simulink model "Biped_Model"  (R2019a)
settings: Solver=VariableStepAuto  StartTime=0.0  StopTime=Time(end)  FixedStep=.001  EnableMultiTasking=on
PreLoadFcn:
  | YBT_HomeDir = pwd;
  | 
  | % Code to use copy within this repository
  | addpath([YBT_HomeDir filesep 'Libraries' filesep 'CFL_Libs']);
  | startup_Contact_Forces
  | 
  | cd(YBT_HomeDir)
  | addpath(YBT_HomeDir);
  | addpath([YBT_HomeDir filesep 'Libraries']);
  | addpath([YBT_HomeDir filesep 'Images']);
  | 
  | Robot_Parameters
model workspace: external: MATLAB File C:\Users\nozaripo\Desktop\BipedalWalking_Simulink_ModelnData\Robot_Parameters.m (data not in the file)
values from neighbouring files (symbols this model uses):
  ankle_servo_kd = 4    [Robot_Parameters.m]
  ankle_servo_ki = 0    [Robot_Parameters.m]
  ankle_servo_kp = 70    [Robot_Parameters.m]
  ankle_to_midLow = 19    [Robot_Parameters.m]
  contact_damping = 50    [Robot_Parameters.m]
  contact_point_radius = 0.005    [Robot_Parameters.m]
  contact_stiffness = 90311    [Robot_Parameters.m]
  deriv_filter_coeff = 50    [Robot_Parameters.m]
  foot_mass = 1    [Robot_Parameters.m]
  height_plane = 0.1    [Robot_Parameters.m]
  hip_servo_kd = 30    [Robot_Parameters.m]
  hip_servo_ki = 0    [Robot_Parameters.m]
  hip_servo_kp = 300    [Robot_Parameters.m]
  init = -joint_angles(1,:)    [Script_Data.m]
  init_vel = -vel(1,:)    [Script_Data.m]
  joint_angles = joint_angles(:,end:-1:1)    [Script_Data.m]
  joint_damping = 0    [Robot_Parameters.m]
  joint_stiffness = 0    [Robot_Parameters.m]
  knee_servo_kd = 30    [Robot_Parameters.m]
  knee_servo_ki = 0    [Robot_Parameters.m]
  knee_servo_kp = 150    [Robot_Parameters.m]
  knee_to_midUpp = 19    [Robot_Parameters.m]
  linear_contact_flag = 0    [Robot_Parameters.m]
  lower_leg_CM_offset = 2.55    [Robot_Parameters.m]
  lower_leg_mass = 2.87    [Robot_Parameters.m]
  max_torque_ank = 45    [Robot_Parameters.m]
  max_torque_hip = 25    [Robot_Parameters.m]
  max_torque_kn = 30    [Robot_Parameters.m]
  midLow_to_knee = 19    [Robot_Parameters.m]
  midUpp_to_hip = 19    [Robot_Parameters.m]
  motion_time_constant = 0.01    [Robot_Parameters.m]
  motor_constant = 0.01    [Robot_Parameters.m]
  motor_inertia = 0    [Robot_Parameters.m]
  mu_k = 0.5    [Robot_Parameters.m]
  mu_s = 0.8    [Robot_Parameters.m]
  mu_vth = 0.1    [Robot_Parameters.m]
  pen_exp = 1.5    [Robot_Parameters.m]
  plane_x = 3    [Robot_Parameters.m]
  plane_y = 0.3    [Robot_Parameters.m]
  split_belt = 0    [Script_Data.m]
  Time = (0:.01:.01*209)'    [Script_Data.m]
  torso_mass = 27.17    [Robot_Parameters.m]
  torso_to_hip = 11    [Robot_Parameters.m]
  upper_leg_CM_offset = 2.55    [Robot_Parameters.m]
  upper_leg_length = 38    [Robot_Parameters.m]
  upper_leg_mass = 4.7    [Robot_Parameters.m]
  V_treadmill = -1.0    (= -1)    [Script_Data.m]
  YBT_Par = struct    [Robot_Parameters.m]
undefined symbols (not defined in the file or in its folder): Extr_Data_LinkHoles, X, Y, Z
libraries: nesl_utility x198, sm_lib x144, fl_lib x42, simulink x20, ee_lib x18, Contact_Forces_Lib x16, Parts_Lib x10, Multibody_Multiphysics_Lib x6, simulink_extras x1
(part 11 of 11)

== system Biped_Model/Robot/Robot Leg L/Box to Belt In Force1/Sphere to Plane Force Enabled nz1/Forces/Force Law ==
  note: 1) Only subsystems can be added as variant choices at this level
      | 2) Blocks cannot be connected at this level as connectivity is
      | automatically determined at simulation, based on the active variant
  Pen : Inport
  Pen Vel : Inport  Port=2
  Custom : Subsystem  VariantControl=Custom  mask(Custom Force Law){k_pen=k_contact, b_penvel=b_contact, cust_param_1=custom_param_1, cust_param_2=custom_param_2}
      mask prompts: k_pen "Contact Stiffness"; b_penvel "Contact Damping"; cust_param_1 "Custom Parameter 1"; cust_param_2 "Custom Parameter 2"
      mask help: This subsystem is for prototyping a custom force law. You can create your own force law in this subsystem and use it in the contact force models in this library by selecting the "Custom" option for the Force Law parameter.
  Linear : Subsystem  VariantControl=Linear  mask(Linear Force Law){k_pen=k_contact, b_penvel=b_contact}
      mask prompts: k_pen "Contact Stiffness"; b_penvel "Contact Damping"
      mask help: Implements a contact force law as a linear spring damper. The damping force is applied only as the penetration depth increases.
      mask Help: web(which('Force_Laws.html'));
  Nonlinear : Subsystem  VariantControl=Nonlinear  mask(Nonlinear Force Law){k_pen=k_contact, b_penvel=b_contact, pen_full_damping=pen_full_damp_F, pen_exp=pen_exponent}
      mask prompts: k_pen "Contact Stiffness"; b_penvel "Contact Damping"; pen_full_damping "Penetration for Full Damping"; pen_exp "Penetration Exponent (>=1)"
      mask help: Implements a contact force law as a nonlinear spring damper. The spring force increases exponentially with penetration. The damping force is multiplied by a scaling factor which is dependent upon the penetration. The scaling factor increases from 0 to 1 as a smooth polynomial until the penetration reaches the value specified by the parameter Penetration for Full Damping. The damping force is applied only as the penetration depth increases.
      mask Help: web(which('Force_Laws.html'));
  Spr F : Outport
  Damp F : Outport  Port=2

== system Biped_Model/Robot/Robot Leg L/Box to Belt In Force1/Sphere to Plane Force Enabled nz2/Forces/Calculate Penetration ==
  z : Inport
  vz : Inport  Port=2
  Abs : Abs  ZeroCross=off
  Constant : Constant  Value=sphere_rad+plane_depth
  Dead Zone : DeadZone  LowerValue=-inf  UpperValue=0  SaturateOnIntegerOverflow=on
  Gain2 : Gain  Gain=-1
  Product : Product
  Sign vx : Signum  ZeroCross=off
  Sign x : Signum  ZeroCross=off
  Sum : Sum  Inputs=+-
  Pos Sign : Outport
  Pen : Outport  Port=2
  Pen Vel : Outport  Port=3
  Vel Sign : Outport  Port=4
  wires:
  Gain2/1 -> Pen Vel/1
  Dead Zone/1 -> Pen/1
  Product/1 -> Gain2/1
  Sign vx/1 -> Vel Sign/1
  Sign x/1 -> Product/1, Pos Sign/1
  Abs/1 -> Sum/2
  Sum/1 -> Dead Zone/1
  Constant/1 -> Sum/1
  vz/1 -> Sign vx/1, Product/2
  z/1 -> Abs/1, Sign x/1

== system Biped_Model/Robot/Robot Leg L/Box to Belt In Force1/Sphere to Plane Force Enabled nz2/Forces/Ff ==
  Fn : Inport
  R : Inport  Port=2
  zSign : Inport  Port=3
  wx : Inport  Port=4
  wy : Inport  Port=5
  vx : Inport  Port=6
  vy : Inport  Port=7
  Cross Product : Contact_Forces_Lib/Math/Cross Product  SystemSampleTime=-1
      settings: SourceProductName=Simscape Multibody Contact Forces Library
  Friction Law : Contact_Forces_Lib/Friction Law  SystemSampleTime=-1  LabelModeActiveChoice=Stick_Slip_C
      settings: SourceProductName=Simscape Multibody Contact Forces Library
  Fx1 : Constant  Value=0
  Fx2 : Constant  Value=[0 0 -sphere_rad]
  Gain : Gain  Gain=-1
  Mux1 : Mux  Inputs=3
  Product1 : Product  Inputs=/*  Multiplication=Matrix(*)
  Product2 : Product  Inputs=/*  Multiplication=Matrix(*)
  Product{3..7} (5 alike) : Product
  Selector : Selector  InputPortWidth=3  IndexOptions=Index vector (dialog)  Indices=3  OutputSizes=1
  SlipVel : Subsystem
  Trigonometric Function : Trigonometry
  Trigonometric Function1 : Trigonometry  Operator=cos
  zSign1 : InportShadow  Port=3
  Ff Sph : Outport
  T Sph : Outport  Port=2
  Ff Pla : Outport  Port=3
  wires:
  Product7/1 -> Cross Product/1
  zSign1/1 -> Product7/2
  Product6/1 -> SlipVel/3(vx)
  zSign/1 -> Product6/2, Product5/1
  Product5/1 -> SlipVel/4(vy)
  Fx2/1 -> Product7/1
  R/1 -> Product2/1, Product1/1
  Cross Product/1 -> Product2/2
  Product1/1 -> Ff Sph/1
  Mux1/1 -> Product1/2, Cross Product/2, Gain/1
  Product2/1 -> T Sph/1
  vy/1 -> Product5/2
  wy/1 -> SlipVel/2(wy)
  wx/1 -> SlipVel/1(wx)
  vx/1 -> Product6/1
  Trigonometric Function/1 -> Product4/2
  Fx1/1 -> Mux1/3
  Product3/1 -> Mux1/1
  Product4/1 -> Mux1/2
  Friction Law/1 -> Product4/1, Product3/1
  Selector/1 -> Friction Law/1
  SlipVel/1(vabs) -> Friction Law/2
  Trigonometric Function1/1 -> Product3/2
  SlipVel/2(alpha) -> Trigonometric Function1/1, Trigonometric Function/1
  Gain/1 -> Ff Pla/1
  Fn/1 -> Selector/1

== system Biped_Model/Robot/Robot Leg L/Box to Belt In Force1/Sphere to Plane Force Enabled nz2/Forces/Fn ==
  R : Inport
  SprF : Inport  Port=2
  DamF : Inport  Port=3
  Fx : Constant  Value=0
  Gain : Gain  Gain=-1
  Mux : Mux  Inputs=3
  Product2 : Product  Inputs=/*  Multiplication=Matrix(*)
  Sum : Sum
  Fn : Outport
  FnF : Outport  Port=2
  FnB : Outport  Port=3
  wires:
  SprF/1 -> Sum/1
  DamF/1 -> Sum/2
  Sum/1 -> Mux/3, Fn/1
  Fx/1 -> Mux/2, Mux/1
  R/1 -> Product2/1
  Gain/1 -> FnB/1
  Product2/1 -> FnF/1
  Mux/1 -> Product2/2, Gain/1

== system Biped_Model/Robot/Robot Leg L/Box to Belt In Force1/Sphere to Plane Force Enabled nz2/Forces/Force Law ==
  note: 1) Only subsystems can be added as variant choices at this level
      | 2) Blocks cannot be connected at this level as connectivity is
      | automatically determined at simulation, based on the active variant
  Pen : Inport
  Pen Vel : Inport  Port=2
  Custom : Subsystem  VariantControl=Custom  mask(Custom Force Law){k_pen=k_contact, b_penvel=b_contact, cust_param_1=custom_param_1, cust_param_2=custom_param_2}
      mask prompts: k_pen "Contact Stiffness"; b_penvel "Contact Damping"; cust_param_1 "Custom Parameter 1"; cust_param_2 "Custom Parameter 2"
      mask help: This subsystem is for prototyping a custom force law. You can create your own force law in this subsystem and use it in the contact force models in this library by selecting the "Custom" option for the Force Law parameter.
  Linear : Subsystem  VariantControl=Linear  mask(Linear Force Law){k_pen=k_contact, b_penvel=b_contact}
      mask prompts: k_pen "Contact Stiffness"; b_penvel "Contact Damping"
      mask help: Implements a contact force law as a linear spring damper. The damping force is applied only as the penetration depth increases.
      mask Help: web(which('Force_Laws.html'));
  Nonlinear : Subsystem  VariantControl=Nonlinear  mask(Nonlinear Force Law){k_pen=k_contact, b_penvel=b_contact, pen_full_damping=pen_full_damp_F, pen_exp=pen_exponent}
      mask prompts: k_pen "Contact Stiffness"; b_penvel "Contact Damping"; pen_full_damping "Penetration for Full Damping"; pen_exp "Penetration Exponent (>=1)"
      mask help: Implements a contact force law as a nonlinear spring damper. The spring force increases exponentially with penetration. The damping force is multiplied by a scaling factor which is dependent upon the penetration. The scaling factor increases from 0 to 1 as a smooth polynomial until the penetration reaches the value specified by the parameter Penetration for Full Damping. The damping force is applied only as the penetration depth increases.
      mask Help: web(which('Force_Laws.html'));
  Spr F : Outport
  Damp F : Outport  Port=2

== system Biped_Model/Robot/Robot Leg R/Box to Belt In Force/Sphere to Plane Force Enabled nz1/Forces/Calculate Penetration ==
  z : Inport
  vz : Inport  Port=2
  Abs : Abs  ZeroCross=off
  Constant : Constant  Value=sphere_rad+plane_depth
  Dead Zone : DeadZone  LowerValue=-inf  UpperValue=0  SaturateOnIntegerOverflow=on
  Gain2 : Gain  Gain=-1
  Product : Product
  Sign vx : Signum  ZeroCross=off
  Sign x : Signum  ZeroCross=off
  Sum : Sum  Inputs=+-
  Pos Sign : Outport
  Pen : Outport  Port=2
  Pen Vel : Outport  Port=3
  Vel Sign : Outport  Port=4
  wires:
  z/1 -> Sign x/1, Abs/1
  vz/1 -> Product/2, Sign vx/1
  Constant/1 -> Sum/1
  Sum/1 -> Dead Zone/1
  Abs/1 -> Sum/2
  Sign x/1 -> Pos Sign/1, Product/1
  Sign vx/1 -> Vel Sign/1
  Product/1 -> Gain2/1
  Dead Zone/1 -> Pen/1
  Gain2/1 -> Pen Vel/1

== system Biped_Model/Robot/Robot Leg R/Box to Belt In Force/Sphere to Plane Force Enabled nz1/Forces/Ff ==
  Fn : Inport
  R : Inport  Port=2
  zSign : Inport  Port=3
  wx : Inport  Port=4
  wy : Inport  Port=5
  vx : Inport  Port=6
  vy : Inport  Port=7
  Cross Product : Contact_Forces_Lib/Math/Cross Product  SystemSampleTime=-1
      settings: SourceProductName=Simscape Multibody Contact Forces Library
  Friction Law : Contact_Forces_Lib/Friction Law  SystemSampleTime=-1  LabelModeActiveChoice=Stick_Slip_C
      settings: SourceProductName=Simscape Multibody Contact Forces Library
  Fx1 : Constant  Value=0
  Fx2 : Constant  Value=[0 0 -sphere_rad]
  Gain : Gain  Gain=-1
  Mux1 : Mux  Inputs=3
  Product1 : Product  Inputs=/*  Multiplication=Matrix(*)
  Product2 : Product  Inputs=/*  Multiplication=Matrix(*)
  Product{3..7} (5 alike) : Product
  Selector : Selector  InputPortWidth=3  IndexOptions=Index vector (dialog)  Indices=3  OutputSizes=1
  SlipVel : Subsystem
  Trigonometric Function : Trigonometry
  Trigonometric Function1 : Trigonometry  Operator=cos
  zSign1 : InportShadow  Port=3
  Ff Sph : Outport
  T Sph : Outport  Port=2
  Ff Pla : Outport  Port=3
  wires:
  Fn/1 -> Selector/1
  Gain/1 -> Ff Pla/1
  SlipVel/2(alpha) -> Trigonometric Function/1, Trigonometric Function1/1
  Trigonometric Function1/1 -> Product3/2
  SlipVel/1(vabs) -> Friction Law/2
  Selector/1 -> Friction Law/1
  Friction Law/1 -> Product3/1, Product4/1
  Product4/1 -> Mux1/2
  Product3/1 -> Mux1/1
  Fx1/1 -> Mux1/3
  Trigonometric Function/1 -> Product4/2
  vx/1 -> Product6/1
  wx/1 -> SlipVel/1(wx)
  wy/1 -> SlipVel/2(wy)
  vy/1 -> Product5/2
  Product2/1 -> T Sph/1
  Mux1/1 -> Gain/1, Cross Product/2, Product1/2
  Product1/1 -> Ff Sph/1
  Cross Product/1 -> Product2/2
  R/1 -> Product1/1, Product2/1
  Fx2/1 -> Product7/1
  Product5/1 -> SlipVel/4(vy)
  zSign/1 -> Product5/1, Product6/2
  Product6/1 -> SlipVel/3(vx)
  zSign1/1 -> Product7/2
  Product7/1 -> Cross Product/1

== system Biped_Model/Robot/Robot Leg R/Box to Belt In Force/Sphere to Plane Force Enabled nz1/Forces/Fn ==
  R : Inport
  SprF : Inport  Port=2
  DamF : Inport  Port=3
  Fx : Constant  Value=0
  Gain : Gain  Gain=-1
  Mux : Mux  Inputs=3
  Product2 : Product  Inputs=/*  Multiplication=Matrix(*)
  Sum : Sum
  Fn : Outport
  FnF : Outport  Port=2
  FnB : Outport  Port=3
  wires:
  Mux/1 -> Gain/1, Product2/2
  Product2/1 -> FnF/1
  Gain/1 -> FnB/1
  R/1 -> Product2/1
  Fx/1 -> Mux/1, Mux/2
  Sum/1 -> Fn/1, Mux/3
  DamF/1 -> Sum/2
  SprF/1 -> Sum/1

== system Biped_Model/Robot/Robot Leg R/Box to Belt In Force/Sphere to Plane Force Enabled nz1/Forces/Force Law ==
  note: 1) Only subsystems can be added as variant choices at this level
      | 2) Blocks cannot be connected at this level as connectivity is
      | automatically determined at simulation, based on the active variant
  Pen : Inport
  Pen Vel : Inport  Port=2
  Custom : Subsystem  VariantControl=Custom  mask(Custom Force Law){k_pen=k_contact, b_penvel=b_contact, cust_param_1=custom_param_1, cust_param_2=custom_param_2}
      mask prompts: k_pen "Contact Stiffness"; b_penvel "Contact Damping"; cust_param_1 "Custom Parameter 1"; cust_param_2 "Custom Parameter 2"
      mask help: This subsystem is for prototyping a custom force law. You can create your own force law in this subsystem and use it in the contact force models in this library by selecting the "Custom" option for the Force Law parameter.
  Linear : Subsystem  VariantControl=Linear  mask(Linear Force Law){k_pen=k_contact, b_penvel=b_contact}
      mask prompts: k_pen "Contact Stiffness"; b_penvel "Contact Damping"
      mask help: Implements a contact force law as a linear spring damper. The damping force is applied only as the penetration depth increases.
      mask Help: web(which('Force_Laws.html'));
  Nonlinear : Subsystem  VariantControl=Nonlinear  mask(Nonlinear Force Law){k_pen=k_contact, b_penvel=b_contact, pen_full_damping=pen_full_damp_F, pen_exp=pen_exponent}
      mask prompts: k_pen "Contact Stiffness"; b_penvel "Contact Damping"; pen_full_damping "Penetration for Full Damping"; pen_exp "Penetration Exponent (>=1)"
      mask help: Implements a contact force law as a nonlinear spring damper. The spring force increases exponentially with penetration. The damping force is multiplied by a scaling factor which is dependent upon the penetration. The scaling factor increases from 0 to 1 as a smooth polynomial until the penetration reaches the value specified by the parameter Penetration for Full Damping. The damping force is applied only as the penetration depth increases.
      mask Help: web(which('Force_Laws.html'));
  Spr F : Outport
  Damp F : Outport  Port=2

== system Biped_Model/Robot/Robot Leg R/Box to Belt In Force/Sphere to Plane Force Enabled nz2/Forces/Calculate Penetration ==
  z : Inport
  vz : Inport  Port=2
  Abs : Abs  ZeroCross=off
  Constant : Constant  Value=sphere_rad+plane_depth
  Dead Zone : DeadZone  LowerValue=-inf  UpperValue=0  SaturateOnIntegerOverflow=on
  Gain2 : Gain  Gain=-1
  Product : Product
  Sign vx : Signum  ZeroCross=off
  Sign x : Signum  ZeroCross=off
  Sum : Sum  Inputs=+-
  Pos Sign : Outport
  Pen : Outport  Port=2
  Pen Vel : Outport  Port=3
  Vel Sign : Outport  Port=4
  wires:
  z/1 -> Sign x/1, Abs/1
  vz/1 -> Product/2, Sign vx/1
  Constant/1 -> Sum/1
  Sum/1 -> Dead Zone/1
  Abs/1 -> Sum/2
  Sign x/1 -> Pos Sign/1, Product/1
  Sign vx/1 -> Vel Sign/1
  Product/1 -> Gain2/1
  Dead Zone/1 -> Pen/1
  Gain2/1 -> Pen Vel/1

== system Biped_Model/Robot/Robot Leg R/Box to Belt In Force/Sphere to Plane Force Enabled nz2/Forces/Ff ==
  Fn : Inport
  R : Inport  Port=2
  zSign : Inport  Port=3
  wx : Inport  Port=4
  wy : Inport  Port=5
  vx : Inport  Port=6
  vy : Inport  Port=7
  Cross Product : Contact_Forces_Lib/Math/Cross Product  SystemSampleTime=-1
      settings: SourceProductName=Simscape Multibody Contact Forces Library
  Friction Law : Contact_Forces_Lib/Friction Law  SystemSampleTime=-1  LabelModeActiveChoice=Stick_Slip_C
      settings: SourceProductName=Simscape Multibody Contact Forces Library
  Fx1 : Constant  Value=0
  Fx2 : Constant  Value=[0 0 -sphere_rad]
  Gain : Gain  Gain=-1
  Mux1 : Mux  Inputs=3
  Product1 : Product  Inputs=/*  Multiplication=Matrix(*)
  Product2 : Product  Inputs=/*  Multiplication=Matrix(*)
  Product{3..7} (5 alike) : Product
  Selector : Selector  InputPortWidth=3  IndexOptions=Index vector (dialog)  Indices=3  OutputSizes=1
  SlipVel : Subsystem
  Trigonometric Function : Trigonometry
  Trigonometric Function1 : Trigonometry  Operator=cos
  zSign1 : InportShadow  Port=3
  Ff Sph : Outport
  T Sph : Outport  Port=2
  Ff Pla : Outport  Port=3
  wires:
  Fn/1 -> Selector/1
  Gain/1 -> Ff Pla/1
  SlipVel/2(alpha) -> Trigonometric Function/1, Trigonometric Function1/1
  Trigonometric Function1/1 -> Product3/2
  SlipVel/1(vabs) -> Friction Law/2
  Selector/1 -> Friction Law/1
  Friction Law/1 -> Product3/1, Product4/1
  Product4/1 -> Mux1/2
  Product3/1 -> Mux1/1
  Fx1/1 -> Mux1/3
  Trigonometric Function/1 -> Product4/2
  vx/1 -> Product6/1
  wx/1 -> SlipVel/1(wx)
  wy/1 -> SlipVel/2(wy)
  vy/1 -> Product5/2
  Product2/1 -> T Sph/1
  Mux1/1 -> Gain/1, Cross Product/2, Product1/2
  Product1/1 -> Ff Sph/1
  Cross Product/1 -> Product2/2
  R/1 -> Product1/1, Product2/1
  Fx2/1 -> Product7/1
  Product5/1 -> SlipVel/4(vy)
  zSign/1 -> Product5/1, Product6/2
  Product6/1 -> SlipVel/3(vx)
  zSign1/1 -> Product7/2
  Product7/1 -> Cross Product/1

== system Biped_Model/Robot/Robot Leg R/Box to Belt In Force/Sphere to Plane Force Enabled nz2/Forces/Fn ==
  R : Inport
  SprF : Inport  Port=2
  DamF : Inport  Port=3
  Fx : Constant  Value=0
  Gain : Gain  Gain=-1
  Mux : Mux  Inputs=3
  Product2 : Product  Inputs=/*  Multiplication=Matrix(*)
  Sum : Sum
  Fn : Outport
  FnF : Outport  Port=2
  FnB : Outport  Port=3
  wires:
  Mux/1 -> Gain/1, Product2/2
  Product2/1 -> FnF/1
  Gain/1 -> FnB/1
  R/1 -> Product2/1
  Fx/1 -> Mux/1, Mux/2
  Sum/1 -> Fn/1, Mux/3
  DamF/1 -> Sum/2
  SprF/1 -> Sum/1

== system Biped_Model/Robot/Robot Leg R/Box to Belt In Force/Sphere to Plane Force Enabled nz2/Forces/Force Law ==
  note: 1) Only subsystems can be added as variant choices at this level
      | 2) Blocks cannot be connected at this level as connectivity is
      | automatically determined at simulation, based on the active variant
  Pen : Inport
  Pen Vel : Inport  Port=2
  Custom : Subsystem  VariantControl=Custom  mask(Custom Force Law){k_pen=k_contact, b_penvel=b_contact, cust_param_1=custom_param_1, cust_param_2=custom_param_2}
      mask prompts: k_pen "Contact Stiffness"; b_penvel "Contact Damping"; cust_param_1 "Custom Parameter 1"; cust_param_2 "Custom Parameter 2"
      mask help: This subsystem is for prototyping a custom force law. You can create your own force law in this subsystem and use it in the contact force models in this library by selecting the "Custom" option for the Force Law parameter.
  Linear : Subsystem  VariantControl=Linear  mask(Linear Force Law){k_pen=k_contact, b_penvel=b_contact}
      mask prompts: k_pen "Contact Stiffness"; b_penvel "Contact Damping"
      mask help: Implements a contact force law as a linear spring damper. The damping force is applied only as the penetration depth increases.
      mask Help: web(which('Force_Laws.html'));
  Nonlinear : Subsystem  VariantControl=Nonlinear  mask(Nonlinear Force Law){k_pen=k_contact, b_penvel=b_contact, pen_full_damping=pen_full_damp_F, pen_exp=pen_exponent}
      mask prompts: k_pen "Contact Stiffness"; b_penvel "Contact Damping"; pen_full_damping "Penetration for Full Damping"; pen_exp "Penetration Exponent (>=1)"
      mask help: Implements a contact force law as a nonlinear spring damper. The spring force increases exponentially with penetration. The damping force is multiplied by a scaling factor which is dependent upon the penetration. The scaling factor increases from 0 to 1 as a smooth polynomial until the penetration reaches the value specified by the parameter Penetration for Full Damping. The damping force is applied only as the penetration depth increases.
      mask Help: web(which('Force_Laws.html'));
  Spr F : Outport
  Damp F : Outport  Port=2

== system Biped_Model/Robot/Robot Leg L/Box to Belt In Force1/Sphere to Plane Force Enabled nz1/Forces/Ff/SlipVel ==
  wx : Inport
  wy : Inport  Port=2
  vx : Inport  Port=3
  vy : Inport  Port=4
  Fx1 : Constant  Value=sphere_rad
  Math Function : Math  Operator=square  SaturateOnIntegerOverflow=on
  Math Function1 : Math  Operator=square  SaturateOnIntegerOverflow=on
  Product3 : Product
  Product4 : Product
  Sqrt : Sqrt  SaturateOnIntegerOverflow=on
  Sum1 : Sum  Inputs=|++
  Sum2 : Sum  Inputs=|-+
  Sum3 : Sum  Inputs=|++
  Trigonometric Function : Trigonometry  Operator=atan2
  vabs : Outport
  alpha : Outport  Port=2
  wires:
  Sum2/1 -> Math Function1/1, Trigonometric Function/2  "slipx"
  Sum1/1 -> Math Function/1, Trigonometric Function/1  "slipy"
  Math Function1/1 -> Sum3/2
  Math Function/1 -> Sum3/1
  Sum3/1 -> Sqrt/1
  Sqrt/1 -> vabs/1
  Trigonometric Function/1 -> alpha/1
  Product4/1 -> Sum2/1
  vy/1 -> Sum1/2
  Fx1/1 -> Product4/1, Product3/2
  vx/1 -> Sum2/2
  wy/1 -> Product4/2
  Product3/1 -> Sum1/1
  wx/1 -> Product3/1

== system Biped_Model/Robot/Robot Leg L/Box to Belt In Force1/Sphere to Plane Force Enabled nz1/Forces/Force Law/Custom ==
  note: Implement your own custom force law in this subsystem.
      | To use it in the contact force models,
      | set the parameter "Force Law" to "Custom".
  Pen : Inport
  Pen Vel : Inport  Port=2
  Abs : Abs  ZeroCross=off
  Gain1 : Gain  Gain=k_pen  Multiplication=Matrix(K*u)  SaturateOnIntegerOverflow=on  OutDataTypeStr=Inherit: Same as input  ParamDataTypeStr=Inherit: Same as input
  Gain2 : Gain  Gain=-b_penvel  Multiplication=Matrix(K*u)  SaturateOnIntegerOverflow=on  OutDataTypeStr=Inherit: Same as input  ParamDataTypeStr=Inherit: Same as input
  Product : Product  RndMeth=Zero
  Saturation : Saturate  UpperLimit=Inf  LowerLimit=0  ZeroCross=off
  Sign : Signum  ZeroCross=off
  Spr F : Outport
  Damp F : Outport  Port=2
  wires:
  Saturation/1 -> Gain2/1
  Pen/1 -> Sign/1, Gain1/1  "Penetration"
  Abs/1 -> Product/1  "Damping_Force_Enable"
  Product/1 -> Damp F/1  "Damping_Force"
  Sign/1 -> Abs/1
  Pen Vel/1 -> Saturation/1  "Pen Vel"
  Gain2/1 -> Product/2  "Damping_Force"
  Gain1/1 -> Spr F/1  "Stiffness_Force"

== system Biped_Model/Robot/Robot Leg L/Box to Belt In Force1/Sphere to Plane Force Enabled nz1/Forces/Force Law/Linear ==
  Pen : Inport
  Pen Vel : Inport  Port=2
  Constant : Constant  Value=pen_exp
  Gain1 : Gain  Gain=k_pen  Multiplication=Matrix(K*u)  SaturateOnIntegerOverflow=on  OutDataTypeStr=Inherit: Same as input  ParamDataTypeStr=Inherit: Same as input
  Gain2 : Gain  Gain=-b_penvel*1.5  Multiplication=Matrix(K*u)  SaturateOnIntegerOverflow=on  OutDataTypeStr=Inherit: Same as input  ParamDataTypeStr=Inherit: Same as input
  Math Function : Math  Operator=pow  SaturateOnIntegerOverflow=on
  Product1 : Product  RndMeth=Zero
  Saturation : Saturate  UpperLimit=Inf  LowerLimit=0  ZeroCross=off
  Spr F : Outport
  Damp F : Outport  Port=2
  wires:
  Pen/1 -> Math Function/1  "Penetration"
  Gain1/1 -> Product1/1, Spr F/1  "Stiffness_Force"
  Pen Vel/1 -> Saturation/1  "Penetration_Velocity"
  Gain2/1 -> Product1/2  "Damping_Force"
  Product1/1 -> Damp F/1
  Saturation/1 -> Gain2/1
  Constant/1 -> Math Function/2
  Math Function/1 -> Gain1/1

== system Biped_Model/Robot/Robot Leg L/Box to Belt In Force1/Sphere to Plane Force Enabled nz1/Forces/Force Law/Nonlinear ==
  Pen : Inport
  Pen Vel : Inport  Port=2
  Constant : Constant  Value=pen_exp
  Gain1 : Gain  Gain=k_pen  Multiplication=Matrix(K*u)  SaturateOnIntegerOverflow=on  OutDataTypeStr=Inherit: Same as input  ParamDataTypeStr=Inherit: Same as input
  Gain2 : Gain  Gain=-b_penvel  Multiplication=Matrix(K*u)  SaturateOnIntegerOverflow=on  OutDataTypeStr=Inherit: Same as input  ParamDataTypeStr=Inherit: Same as input
  Math Function : Math  Operator=pow  SaturateOnIntegerOverflow=on
  Product1 : Product  RndMeth=Zero
  Saturation : Saturate  UpperLimit=Inf  LowerLimit=0  ZeroCross=off
  Smoothstep : Subsystem  mask{min_out=0, max_out=1, step_start=0, step_finish=pen_full_damping}
      mask prompts: min_out "Minimum output"; max_out "Maximum output"; step_start "Start Step"; step_finish "Finish Step"
  Spr F : Outport
  Damp F : Outport  Port=2
  wires:
  Saturation/1 -> Gain2/1
  Product1/1 -> Damp F/1
  Smoothstep/1(Out1) -> Product1/1  "Damping_Enable"
  Gain2/1 -> Product1/2  "Damping_Force"
  Constant/1 -> Math Function/2
  Math Function/1 -> Gain1/1
  Pen/1 -> Math Function/1, Smoothstep/1(In1)  "Penetration"
  Pen Vel/1 -> Saturation/1  "Penetration_Velocity"
  Gain1/1 -> Spr F/1  "Stiffness_Force"

== system Biped_Model/Robot/Robot Leg L/Box to Belt In Force1/Sphere to Plane Force Enabled nz2/Forces/Ff/SlipVel ==
  wx : Inport
  wy : Inport  Port=2
  vx : Inport  Port=3
  vy : Inport  Port=4
  Fx1 : Constant  Value=sphere_rad
  Math Function : Math  Operator=square  SaturateOnIntegerOverflow=on
  Math Function1 : Math  Operator=square  SaturateOnIntegerOverflow=on
  Product3 : Product
  Product4 : Product
  Sqrt : Sqrt  SaturateOnIntegerOverflow=on
  Sum1 : Sum  Inputs=|++
  Sum2 : Sum  Inputs=|-+
  Sum3 : Sum  Inputs=|++
  Trigonometric Function : Trigonometry  Operator=atan2
  vabs : Outport
  alpha : Outport  Port=2
  wires:
  wx/1 -> Product3/1
  Product3/1 -> Sum1/1
  wy/1 -> Product4/2
  vx/1 -> Sum2/2
  Fx1/1 -> Product3/2, Product4/1
  vy/1 -> Sum1/2
  Product4/1 -> Sum2/1
  Trigonometric Function/1 -> alpha/1
  Sqrt/1 -> vabs/1
  Sum3/1 -> Sqrt/1
  Math Function/1 -> Sum3/1
  Math Function1/1 -> Sum3/2
  Sum1/1 -> Trigonometric Function/1, Math Function/1  "slipy"
  Sum2/1 -> Trigonometric Function/2, Math Function1/1  "slipx"

== system Biped_Model/Robot/Robot Leg L/Box to Belt In Force1/Sphere to Plane Force Enabled nz2/Forces/Force Law/Custom ==
  note: Implement your own custom force law in this subsystem.
      | To use it in the contact force models,
      | set the parameter "Force Law" to "Custom".
  Pen : Inport
  Pen Vel : Inport  Port=2
  Abs : Abs  ZeroCross=off
  Gain1 : Gain  Gain=k_pen  Multiplication=Matrix(K*u)  SaturateOnIntegerOverflow=on  OutDataTypeStr=Inherit: Same as input  ParamDataTypeStr=Inherit: Same as input
  Gain2 : Gain  Gain=-b_penvel  Multiplication=Matrix(K*u)  SaturateOnIntegerOverflow=on  OutDataTypeStr=Inherit: Same as input  ParamDataTypeStr=Inherit: Same as input
  Product : Product  RndMeth=Zero
  Saturation : Saturate  UpperLimit=Inf  LowerLimit=0  ZeroCross=off
  Sign : Signum  ZeroCross=off
  Spr F : Outport
  Damp F : Outport  Port=2
  wires:
  Gain1/1 -> Spr F/1  "Stiffness_Force"
  Gain2/1 -> Product/2  "Damping_Force"
  Pen Vel/1 -> Saturation/1  "Pen Vel"
  Sign/1 -> Abs/1
  Product/1 -> Damp F/1  "Damping_Force"
  Abs/1 -> Product/1  "Damping_Force_Enable"
  Pen/1 -> Gain1/1, Sign/1  "Penetration"
  Saturation/1 -> Gain2/1

== system Biped_Model/Robot/Robot Leg L/Box to Belt In Force1/Sphere to Plane Force Enabled nz2/Forces/Force Law/Linear ==
  Pen : Inport
  Pen Vel : Inport  Port=2
  Constant : Constant  Value=pen_exp
  Gain1 : Gain  Gain=k_pen  Multiplication=Matrix(K*u)  SaturateOnIntegerOverflow=on  OutDataTypeStr=Inherit: Same as input  ParamDataTypeStr=Inherit: Same as input
  Gain2 : Gain  Gain=-b_penvel*1.5  Multiplication=Matrix(K*u)  SaturateOnIntegerOverflow=on  OutDataTypeStr=Inherit: Same as input  ParamDataTypeStr=Inherit: Same as input
  Math Function : Math  Operator=pow  SaturateOnIntegerOverflow=on
  Product1 : Product  RndMeth=Zero
  Saturation : Saturate  UpperLimit=Inf  LowerLimit=0  ZeroCross=off
  Spr F : Outport
  Damp F : Outport  Port=2
  wires:
  Math Function/1 -> Gain1/1
  Constant/1 -> Math Function/2
  Saturation/1 -> Gain2/1
  Product1/1 -> Damp F/1
  Gain2/1 -> Product1/2  "Damping_Force"
  Pen Vel/1 -> Saturation/1  "Penetration_Velocity"
  Gain1/1 -> Spr F/1, Product1/1  "Stiffness_Force"
  Pen/1 -> Math Function/1  "Penetration"

== system Biped_Model/Robot/Robot Leg L/Box to Belt In Force1/Sphere to Plane Force Enabled nz2/Forces/Force Law/Nonlinear ==
  Pen : Inport
  Pen Vel : Inport  Port=2
  Constant : Constant  Value=pen_exp
  Gain1 : Gain  Gain=k_pen  Multiplication=Matrix(K*u)  SaturateOnIntegerOverflow=on  OutDataTypeStr=Inherit: Same as input  ParamDataTypeStr=Inherit: Same as input
  Gain2 : Gain  Gain=-b_penvel  Multiplication=Matrix(K*u)  SaturateOnIntegerOverflow=on  OutDataTypeStr=Inherit: Same as input  ParamDataTypeStr=Inherit: Same as input
  Math Function : Math  Operator=pow  SaturateOnIntegerOverflow=on
  Product1 : Product  RndMeth=Zero
  Saturation : Saturate  UpperLimit=Inf  LowerLimit=0  ZeroCross=off
  Smoothstep : Subsystem  mask{min_out=0, max_out=1, step_start=0, step_finish=pen_full_damping}
      mask prompts: min_out "Minimum output"; max_out "Maximum output"; step_start "Start Step"; step_finish "Finish Step"
  Spr F : Outport
  Damp F : Outport  Port=2
  wires:
  Gain1/1 -> Spr F/1  "Stiffness_Force"
  Pen Vel/1 -> Saturation/1  "Penetration_Velocity"
  Pen/1 -> Smoothstep/1(In1), Math Function/1  "Penetration"
  Math Function/1 -> Gain1/1
  Constant/1 -> Math Function/2
  Gain2/1 -> Product1/2  "Damping_Force"
  Smoothstep/1(Out1) -> Product1/1  "Damping_Enable"
  Product1/1 -> Damp F/1
  Saturation/1 -> Gain2/1

== system Biped_Model/Robot/Robot Leg R/Box to Belt In Force/Sphere to Plane Force Enabled nz1/Forces/Ff/SlipVel ==
  wx : Inport
  wy : Inport  Port=2
  vx : Inport  Port=3
  vy : Inport  Port=4
  Fx1 : Constant  Value=sphere_rad
  Math Function : Math  Operator=square  SaturateOnIntegerOverflow=on
  Math Function1 : Math  Operator=square  SaturateOnIntegerOverflow=on
  Product3 : Product
  Product4 : Product
  Sqrt : Sqrt  SaturateOnIntegerOverflow=on
  Sum1 : Sum  Inputs=|++
  Sum2 : Sum  Inputs=|-+
  Sum3 : Sum  Inputs=|++
  Trigonometric Function : Trigonometry  Operator=atan2
  vabs : Outport
  alpha : Outport  Port=2
  wires:
  Sum2/1 -> Math Function1/1, Trigonometric Function/2  "slipx"
  Sum1/1 -> Math Function/1, Trigonometric Function/1  "slipy"
  Math Function1/1 -> Sum3/2
  Math Function/1 -> Sum3/1
  Sum3/1 -> Sqrt/1
  Sqrt/1 -> vabs/1
  Trigonometric Function/1 -> alpha/1
  Product4/1 -> Sum2/1
  vy/1 -> Sum1/2
  Fx1/1 -> Product4/1, Product3/2
  vx/1 -> Sum2/2
  wy/1 -> Product4/2
  Product3/1 -> Sum1/1
  wx/1 -> Product3/1

== system Biped_Model/Robot/Robot Leg R/Box to Belt In Force/Sphere to Plane Force Enabled nz1/Forces/Force Law/Custom ==
  note: Implement your own custom force law in this subsystem.
      | To use it in the contact force models,
      | set the parameter "Force Law" to "Custom".
  Pen : Inport
  Pen Vel : Inport  Port=2
  Abs : Abs  ZeroCross=off
  Gain1 : Gain  Gain=k_pen  Multiplication=Matrix(K*u)  SaturateOnIntegerOverflow=on  OutDataTypeStr=Inherit: Same as input  ParamDataTypeStr=Inherit: Same as input
  Gain2 : Gain  Gain=-b_penvel  Multiplication=Matrix(K*u)  SaturateOnIntegerOverflow=on  OutDataTypeStr=Inherit: Same as input  ParamDataTypeStr=Inherit: Same as input
  Product : Product  RndMeth=Zero
  Saturation : Saturate  UpperLimit=Inf  LowerLimit=0  ZeroCross=off
  Sign : Signum  ZeroCross=off
  Spr F : Outport
  Damp F : Outport  Port=2
  wires:
  Saturation/1 -> Gain2/1
  Pen/1 -> Sign/1, Gain1/1  "Penetration"
  Abs/1 -> Product/1  "Damping_Force_Enable"
  Product/1 -> Damp F/1  "Damping_Force"
  Sign/1 -> Abs/1
  Pen Vel/1 -> Saturation/1  "Pen Vel"
  Gain2/1 -> Product/2  "Damping_Force"
  Gain1/1 -> Spr F/1  "Stiffness_Force"

== system Biped_Model/Robot/Robot Leg R/Box to Belt In Force/Sphere to Plane Force Enabled nz1/Forces/Force Law/Linear ==
  Pen : Inport
  Pen Vel : Inport  Port=2
  Constant : Constant  Value=pen_exp
  Gain1 : Gain  Gain=k_pen  Multiplication=Matrix(K*u)  SaturateOnIntegerOverflow=on  OutDataTypeStr=Inherit: Same as input  ParamDataTypeStr=Inherit: Same as input
  Gain2 : Gain  Gain=-b_penvel*1.5  Multiplication=Matrix(K*u)  SaturateOnIntegerOverflow=on  OutDataTypeStr=Inherit: Same as input  ParamDataTypeStr=Inherit: Same as input
  Math Function : Math  Operator=pow  SaturateOnIntegerOverflow=on
  Product1 : Product  RndMeth=Zero
  Saturation : Saturate  UpperLimit=Inf  LowerLimit=0  ZeroCross=off
  Spr F : Outport
  Damp F : Outport  Port=2
  wires:
  Pen/1 -> Math Function/1  "Penetration"
  Gain1/1 -> Product1/1, Spr F/1  "Stiffness_Force"
  Pen Vel/1 -> Saturation/1  "Penetration_Velocity"
  Gain2/1 -> Product1/2  "Damping_Force"
  Product1/1 -> Damp F/1
  Saturation/1 -> Gain2/1
  Constant/1 -> Math Function/2
  Math Function/1 -> Gain1/1

== system Biped_Model/Robot/Robot Leg R/Box to Belt In Force/Sphere to Plane Force Enabled nz1/Forces/Force Law/Nonlinear ==
  Pen : Inport
  Pen Vel : Inport  Port=2
  Constant : Constant  Value=pen_exp
  Gain1 : Gain  Gain=k_pen  Multiplication=Matrix(K*u)  SaturateOnIntegerOverflow=on  OutDataTypeStr=Inherit: Same as input  ParamDataTypeStr=Inherit: Same as input
  Gain2 : Gain  Gain=-b_penvel  Multiplication=Matrix(K*u)  SaturateOnIntegerOverflow=on  OutDataTypeStr=Inherit: Same as input  ParamDataTypeStr=Inherit: Same as input
  Math Function : Math  Operator=pow  SaturateOnIntegerOverflow=on
  Product1 : Product  RndMeth=Zero
  Saturation : Saturate  UpperLimit=Inf  LowerLimit=0  ZeroCross=off
  Smoothstep : Subsystem  mask{min_out=0, max_out=1, step_start=0, step_finish=pen_full_damping}
      mask prompts: min_out "Minimum output"; max_out "Maximum output"; step_start "Start Step"; step_finish "Finish Step"
  Spr F : Outport
  Damp F : Outport  Port=2
  wires:
  Saturation/1 -> Gain2/1
  Product1/1 -> Damp F/1
  Smoothstep/1(Out1) -> Product1/1  "Damping_Enable"
  Gain2/1 -> Product1/2  "Damping_Force"
  Constant/1 -> Math Function/2
  Math Function/1 -> Gain1/1
  Pen/1 -> Math Function/1, Smoothstep/1(In1)  "Penetration"
  Pen Vel/1 -> Saturation/1  "Penetration_Velocity"
  Gain1/1 -> Spr F/1  "Stiffness_Force"

== system Biped_Model/Robot/Robot Leg R/Box to Belt In Force/Sphere to Plane Force Enabled nz2/Forces/Ff/SlipVel ==
  wx : Inport
  wy : Inport  Port=2
  vx : Inport  Port=3
  vy : Inport  Port=4
  Fx1 : Constant  Value=sphere_rad
  Math Function : Math  Operator=square  SaturateOnIntegerOverflow=on
  Math Function1 : Math  Operator=square  SaturateOnIntegerOverflow=on
  Product3 : Product
  Product4 : Product
  Sqrt : Sqrt  SaturateOnIntegerOverflow=on
  Sum1 : Sum  Inputs=|++
  Sum2 : Sum  Inputs=|-+
  Sum3 : Sum  Inputs=|++
  Trigonometric Function : Trigonometry  Operator=atan2
  vabs : Outport
  alpha : Outport  Port=2
  wires:
  Sum2/1 -> Math Function1/1, Trigonometric Function/2  "slipx"
  Sum1/1 -> Math Function/1, Trigonometric Function/1  "slipy"
  Math Function1/1 -> Sum3/2
  Math Function/1 -> Sum3/1
  Sum3/1 -> Sqrt/1
  Sqrt/1 -> vabs/1
  Trigonometric Function/1 -> alpha/1
  Product4/1 -> Sum2/1
  vy/1 -> Sum1/2
  Fx1/1 -> Product4/1, Product3/2
  vx/1 -> Sum2/2
  wy/1 -> Product4/2
  Product3/1 -> Sum1/1
  wx/1 -> Product3/1

== system Biped_Model/Robot/Robot Leg R/Box to Belt In Force/Sphere to Plane Force Enabled nz2/Forces/Force Law/Custom ==
  note: Implement your own custom force law in this subsystem.
      | To use it in the contact force models,
      | set the parameter "Force Law" to "Custom".
  Pen : Inport
  Pen Vel : Inport  Port=2
  Abs : Abs  ZeroCross=off
  Gain1 : Gain  Gain=k_pen  Multiplication=Matrix(K*u)  SaturateOnIntegerOverflow=on  OutDataTypeStr=Inherit: Same as input  ParamDataTypeStr=Inherit: Same as input
  Gain2 : Gain  Gain=-b_penvel  Multiplication=Matrix(K*u)  SaturateOnIntegerOverflow=on  OutDataTypeStr=Inherit: Same as input  ParamDataTypeStr=Inherit: Same as input
  Product : Product  RndMeth=Zero
  Saturation : Saturate  UpperLimit=Inf  LowerLimit=0  ZeroCross=off
  Sign : Signum  ZeroCross=off
  Spr F : Outport
  Damp F : Outport  Port=2
  wires:
  Saturation/1 -> Gain2/1
  Pen/1 -> Sign/1, Gain1/1  "Penetration"
  Abs/1 -> Product/1  "Damping_Force_Enable"
  Product/1 -> Damp F/1  "Damping_Force"
  Sign/1 -> Abs/1
  Pen Vel/1 -> Saturation/1  "Pen Vel"
  Gain2/1 -> Product/2  "Damping_Force"
  Gain1/1 -> Spr F/1  "Stiffness_Force"

== system Biped_Model/Robot/Robot Leg R/Box to Belt In Force/Sphere to Plane Force Enabled nz2/Forces/Force Law/Linear ==
  Pen : Inport
  Pen Vel : Inport  Port=2
  Constant : Constant  Value=pen_exp
  Gain1 : Gain  Gain=k_pen  Multiplication=Matrix(K*u)  SaturateOnIntegerOverflow=on  OutDataTypeStr=Inherit: Same as input  ParamDataTypeStr=Inherit: Same as input
  Gain2 : Gain  Gain=-b_penvel*1.5  Multiplication=Matrix(K*u)  SaturateOnIntegerOverflow=on  OutDataTypeStr=Inherit: Same as input  ParamDataTypeStr=Inherit: Same as input
  Math Function : Math  Operator=pow  SaturateOnIntegerOverflow=on
  Product1 : Product  RndMeth=Zero
  Saturation : Saturate  UpperLimit=Inf  LowerLimit=0  ZeroCross=off
  Spr F : Outport
  Damp F : Outport  Port=2
  wires:
  Pen/1 -> Math Function/1  "Penetration"
  Gain1/1 -> Product1/1, Spr F/1  "Stiffness_Force"
  Pen Vel/1 -> Saturation/1  "Penetration_Velocity"
  Gain2/1 -> Product1/2  "Damping_Force"
  Product1/1 -> Damp F/1
  Saturation/1 -> Gain2/1
  Constant/1 -> Math Function/2
  Math Function/1 -> Gain1/1

== system Biped_Model/Robot/Robot Leg R/Box to Belt In Force/Sphere to Plane Force Enabled nz2/Forces/Force Law/Nonlinear ==
  Pen : Inport
  Pen Vel : Inport  Port=2
  Constant : Constant  Value=pen_exp
  Gain1 : Gain  Gain=k_pen  Multiplication=Matrix(K*u)  SaturateOnIntegerOverflow=on  OutDataTypeStr=Inherit: Same as input  ParamDataTypeStr=Inherit: Same as input
  Gain2 : Gain  Gain=-b_penvel  Multiplication=Matrix(K*u)  SaturateOnIntegerOverflow=on  OutDataTypeStr=Inherit: Same as input  ParamDataTypeStr=Inherit: Same as input
  Math Function : Math  Operator=pow  SaturateOnIntegerOverflow=on
  Product1 : Product  RndMeth=Zero
  Saturation : Saturate  UpperLimit=Inf  LowerLimit=0  ZeroCross=off
  Smoothstep : Subsystem  mask{min_out=0, max_out=1, step_start=0, step_finish=pen_full_damping}
      mask prompts: min_out "Minimum output"; max_out "Maximum output"; step_start "Start Step"; step_finish "Finish Step"
  Spr F : Outport
  Damp F : Outport  Port=2
  wires:
  Saturation/1 -> Gain2/1
  Product1/1 -> Damp F/1
  Smoothstep/1(Out1) -> Product1/1  "Damping_Enable"
  Gain2/1 -> Product1/2  "Damping_Force"
  Constant/1 -> Math Function/2
  Math Function/1 -> Gain1/1
  Pen/1 -> Math Function/1, Smoothstep/1(In1)  "Penetration"
  Pen Vel/1 -> Saturation/1  "Penetration_Velocity"
  Gain1/1 -> Spr F/1  "Stiffness_Force"

== system Biped_Model/Robot/Robot Leg L/Box to Belt In Force1/Sphere to Plane Force Enabled nz1/Forces/Force Law/Nonlinear/Smoothstep ==
  In1 : Inport
  Clamp : Saturate  UpperLimit=step_finish  LowerLimit=step_start
  Constant : Constant  Value=3
  Divide : Product  Inputs=*/
  Divide1 : Product  Inputs=****
  Gain : Gain  Gain=2
  Subtract : Sum  Inputs=+-
  Subtract1 : Sum  Inputs=-+
  Subtract2 : Sum
  Subtract3 : Sum  Inputs=+-
  Subtract4 : Sum  Inputs=+-
  max out : Constant  Value=max_out
  min out : Constant  Value=min_out
  step finish : Constant  Value=step_finish
  step start : Constant  Value=step_start
  Out1 : Outport
  wires:
  step start/1 -> Subtract1/1, Subtract/2
  In1/1 -> Clamp/1
  Subtract1/1 -> Divide/2
  Divide/1 -> Gain/1, Divide1/2, Divide1/3
  Subtract/1 -> Divide/1
  Subtract2/1 -> Out1/1
  Constant/1 -> Subtract4/1
  min out/1 -> Subtract2/2, Subtract3/2
  max out/1 -> Subtract3/1
  Clamp/1 -> Subtract/1
  step finish/1 -> Subtract1/2
  Divide1/1 -> Subtract2/1
  Gain/1 -> Subtract4/2
  Subtract4/1 -> Divide1/1
  Subtract3/1 -> Divide1/4

== system Biped_Model/Robot/Robot Leg L/Box to Belt In Force1/Sphere to Plane Force Enabled nz2/Forces/Force Law/Nonlinear/Smoothstep ==
  In1 : Inport
  Clamp : Saturate  UpperLimit=step_finish  LowerLimit=step_start
  Constant : Constant  Value=3
  Divide : Product  Inputs=*/
  Divide1 : Product  Inputs=****
  Gain : Gain  Gain=2
  Subtract : Sum  Inputs=+-
  Subtract1 : Sum  Inputs=-+
  Subtract2 : Sum
  Subtract3 : Sum  Inputs=+-
  Subtract4 : Sum  Inputs=+-
  max out : Constant  Value=max_out
  min out : Constant  Value=min_out
  step finish : Constant  Value=step_finish
  step start : Constant  Value=step_start
  Out1 : Outport
  wires:
  Subtract3/1 -> Divide1/4
  Subtract4/1 -> Divide1/1
  Gain/1 -> Subtract4/2
  Divide1/1 -> Subtract2/1
  step finish/1 -> Subtract1/2
  Clamp/1 -> Subtract/1
  max out/1 -> Subtract3/1
  min out/1 -> Subtract3/2, Subtract2/2
  Constant/1 -> Subtract4/1
  Subtract2/1 -> Out1/1
  Subtract/1 -> Divide/1
  Divide/1 -> Divide1/3, Divide1/2, Gain/1
  Subtract1/1 -> Divide/2
  In1/1 -> Clamp/1
  step start/1 -> Subtract/2, Subtract1/1

== system Biped_Model/Robot/Robot Leg R/Box to Belt In Force/Sphere to Plane Force Enabled nz1/Forces/Force Law/Nonlinear/Smoothstep ==
  In1 : Inport
  Clamp : Saturate  UpperLimit=step_finish  LowerLimit=step_start
  Constant : Constant  Value=3
  Divide : Product  Inputs=*/
  Divide1 : Product  Inputs=****
  Gain : Gain  Gain=2
  Subtract : Sum  Inputs=+-
  Subtract1 : Sum  Inputs=-+
  Subtract2 : Sum
  Subtract3 : Sum  Inputs=+-
  Subtract4 : Sum  Inputs=+-
  max out : Constant  Value=max_out
  min out : Constant  Value=min_out
  step finish : Constant  Value=step_finish
  step start : Constant  Value=step_start
  Out1 : Outport
  wires:
  step start/1 -> Subtract1/1, Subtract/2
  In1/1 -> Clamp/1
  Subtract1/1 -> Divide/2
  Divide/1 -> Gain/1, Divide1/2, Divide1/3
  Subtract/1 -> Divide/1
  Subtract2/1 -> Out1/1
  Constant/1 -> Subtract4/1
  min out/1 -> Subtract2/2, Subtract3/2
  max out/1 -> Subtract3/1
  Clamp/1 -> Subtract/1
  step finish/1 -> Subtract1/2
  Divide1/1 -> Subtract2/1
  Gain/1 -> Subtract4/2
  Subtract4/1 -> Divide1/1
  Subtract3/1 -> Divide1/4

== system Biped_Model/Robot/Robot Leg R/Box to Belt In Force/Sphere to Plane Force Enabled nz2/Forces/Force Law/Nonlinear/Smoothstep ==
  In1 : Inport
  Clamp : Saturate  UpperLimit=step_finish  LowerLimit=step_start
  Constant : Constant  Value=3
  Divide : Product  Inputs=*/
  Divide1 : Product  Inputs=****
  Gain : Gain  Gain=2
  Subtract : Sum  Inputs=+-
  Subtract1 : Sum  Inputs=-+
  Subtract2 : Sum
  Subtract3 : Sum  Inputs=+-
  Subtract4 : Sum  Inputs=+-
  max out : Constant  Value=max_out
  min out : Constant  Value=min_out
  step finish : Constant  Value=step_finish
  step start : Constant  Value=step_start
  Out1 : Outport
  wires:
  step start/1 -> Subtract1/1, Subtract/2
  In1/1 -> Clamp/1
  Subtract1/1 -> Divide/2
  Divide/1 -> Gain/1, Divide1/2, Divide1/3
  Subtract/1 -> Divide/1
  Subtract2/1 -> Out1/1
  Constant/1 -> Subtract4/1
  min out/1 -> Subtract2/2, Subtract3/2
  max out/1 -> Subtract3/1
  Clamp/1 -> Subtract/1
  step finish/1 -> Subtract1/2
  Divide1/1 -> Subtract2/1
  Gain/1 -> Subtract4/2
  Subtract4/1 -> Divide1/1
  Subtract3/1 -> Divide1/4

== matlab function Biped_Model/Robot/Robot Leg R/Box to Belt In Force/Sphere to Plane Force Enabled nz1/MATLAB Function ==
  data: x input; Fx output; y input; z input; vz input; R input; wx input; wy input; vx input; vy input; mu input; Fz output; stiffness input; damping input; pen_exp input; linear_contact_flag input
function [Fx, Fz] = fcn(x, y, z, vz, R, wx, wy, vx, vy, mu, stiffness, damping, pen_exp, linear_contact_flag)

z = z-0.055;
vz= min(vz,0);

if z<=0
    
    if linear_contact_flag ==1
        F_spring = stiffness*(-z);
        F_damper = (-vz)*damping;
    else
        F_spring = stiffness*(-z)^pen_exp;
        F_damper = F_spring*(-vz)*1.5*damping;
    end
    
    Fz = F_spring + F_damper;
    
    Fx = -mu*Fz;
    
else
    Fz = 0;
    Fx = 0;
    
end

== matlab function Biped_Model/Robot/Robot Leg R/Box to Belt In Force/Sphere to Plane Force Enabled nz2/MATLAB Function ==
  data: x input; Fx output; y input; z input; vz input; R input; wx input; wy input; vx input; vy input; mu input; Fz output; stiffness input; damping input; pen_exp input; linear_contact_flag input; F_spring output; F_damper output
function [Fx, Fz, F_spring, F_damper] = fcn(x, y, z, vz, R, wx, wy, vx, vy, mu, stiffness, damping, pen_exp, linear_contact_flag)

z = z-0.055;
vz= min(vz,0);

F_spring = 0;
F_damper = 0;

if z<=0
    
    if linear_contact_flag ==1
        F_spring = stiffness*(-z);
        F_damper = (-vz)*damping;
    else
        F_spring = stiffness*(-z)^pen_exp;
        F_damper = F_spring*(-vz)*1.5*damping;
    end
    
    Fz = F_spring + F_damper;
    
    Fx = -mu*Fz;
    
else
    Fz = 0;
    Fx = 0;
    
end

== matlab function Biped_Model/Robot/Robot Leg L/Box to Belt In Force1/Sphere to Plane Force Enabled nz2/MATLAB Function ==
  data: x input; Fx output; y input; z input; vz input; R input; wx input; wy input; vx input; vy input; mu input; Fz output; stiffness input; damping input; pen_exp input; linear_contact_flag input
function [Fx, Fz] = fcn(x, y, z, vz, R, wx, wy, vx, vy, mu, stiffness, damping, pen_exp, linear_contact_flag)

z = z-0.055;
vz= min(vz,0);

if z<=0
    
    if linear_contact_flag ==1
        F_spring = stiffness*(-z);
        F_damper = (-vz)*damping;
    else
        F_spring = stiffness*(-z)^pen_exp;
        F_damper = F_spring*(-vz)*1.5*damping;
    end
    
    Fz = F_spring + F_damper;
    
    Fx = -mu*Fz;
    
else
    Fz = 0;
    Fx = 0;
    
end

== matlab function Biped_Model/Robot/Robot Leg L/Box to Belt In Force1/Sphere to Plane Force Enabled nz1/MATLAB Function ==
  data: x input; Fx output; y input; z input; vz input; R input; wx input; wy input; vx input; vy input; mu input; Fz output; stiffness input; damping input; pen_exp input; linear_contact_flag input
function [Fx, Fz] = fcn(x, y, z, vz, R, wx, wy, vx, vy, mu, stiffness, damping, pen_exp, linear_contact_flag)

z = z-0.055;
vz= min(vz,0);

if z<=0
    
    if linear_contact_flag ==1
        F_spring = stiffness*(-z);
        F_damper = (-vz)*damping;
    else
        F_spring = stiffness*(-z)^pen_exp;
        F_damper = F_spring*(-vz)*1.5*damping;
    end
    
    
    Fz = F_spring + F_damper;
    
    Fx = -mu*Fz;
    
else
    Fz = 0;
    Fx = 0;
    
end
